simulink model "FX450_model"  (R2019a)
settings: Solver=ode4  StartTime=0.0  StopTime=35  FixedStep=0.001  RelTol=1e-3
PreLoadFcn:
  | filepath  = fileparts(get_param(bdroot, 'FileName'))
  | cd(filepath);
InitFcn:
  | Model_Params;
values from neighbouring files (symbols this model uses):
  aM = 0.478857985732115    (= 0.478857985732)    [Model_Params.m]
  aT = 10.3223    [Model_Params.m]
  bT = 1.7118    [Model_Params.m]
  ModelParam_envAltitude = -50    [Model_Params.m]
  ModelParam_GlobalNoiseGainSwitch = 0.4    [Model_Params.m]
  ModelParam_GPSEphFinal = 0.3    [Model_Params.m]
  ModelParam_GPSEpvFinal = 0.4    [Model_Params.m]
  ModelParam_GPSFix3DFix = 3    [Model_Params.m]
  ModelParam_GPSSatsVisible = 10    [Model_Params.m]
  ModelParam_motorJm = 0    [Model_Params.m]
  ModelParam_noiseBaroCoupleWithSpeed = 0    [Model_Params.m]
  ModelParam_noiseGPSSampTime = 0.2    [Model_Params.m]
  ModelParam_noisePowerIMU = 0    [Model_Params.m]
  ModelParam_noisePowerOffGainAccel = 0.04    [Model_Params.m]
  ModelParam_noisePowerOffGainAccelZ = 0.03    [Model_Params.m]
  ModelParam_noisePowerOffGainGyro = 0.02    [Model_Params.m]
  ModelParam_noisePowerOffGainGyroZ = 0.025    [Model_Params.m]
  ModelParam_noisePowerOffGainMag = 0.02    [Model_Params.m]
  ModelParam_noisePowerOffGainMagZ = 0.035    [Model_Params.m]
  ModelParam_noisePowerOnGainAccel = 0.8    [Model_Params.m]
  ModelParam_noisePowerOnGainAccelZ = 4.5    [Model_Params.m]
  ModelParam_noisePowerOnGainGyro = 2    [Model_Params.m]
  ModelParam_noisePowerOnGainGyroZ = 1    [Model_Params.m]
  ModelParam_noisePowerOnGainMag = 0.025    [Model_Params.m]
  ModelParam_noisePowerOnGainMagZ = 0.05    [Model_Params.m]
  ModelParam_noiseSampleTimeAccel = 0.001    [Model_Params.m]
  ModelParam_noiseSampleTimeGyro = 0.001    [Model_Params.m]
  ModelParam_noiseSampleTimeMag = 0.01    [Model_Params.m]
  ModelParam_noiseUpperGPS = 0.5    [Model_Params.m]
  ModelParam_noiseUpperWindBodyRatio = 0    [Model_Params.m]
  ModelParam_noiseWindSampTime = 0.001    [Model_Params.m]
  ModelParam_timeSampBaro = 0.01    [Model_Params.m]
  ModelParam_uavCCm = [0.0097 0.0085 0.0046]    [Model_Params.m]
  ModelParam_uavCd = [0.2325, 0.2333, 0.5]    [Model_Params.m]
  ModelParam_uavMass = 1.8446    [Model_Params.m]
  ModelParam_uavR = 0.2250    (= 0.225)    [Model_Params.m]
  ModelParam_uavType = int8(3)    [Model_Params.m]
  w1 = -1.813988338293334e+02    (= -181.398833829)    [Model_Params.m]
  w2 = -4.589750663718388e+02    (= -458.975066372)    [Model_Params.m]
  w3 = 1.452124200290536e+03    (= 1452.12420029)    [Model_Params.m]
undefined symbols (not defined in the file or in its folder): Earth, ModelParam_GPSEpvInitial, ModelParam_GPSEpvTimeConstant, ModelParam_noiseLowPassFilterCoeAccel, ModelParam_noiseLowPassFilterCoeGyro, ModelParam_timeSamp, Newton, Raphson, WGS84
libraries: simulink x4, aerolibtransform2 x3, sharedtransform x3, aerolibasang x3, aerolibatmos2 x2, aerolibutil x2, aerolibconvert2 x1, aerolibobsolete x1, shared6dof x1, aerolibnav x1, aerolibgravity2 x1
(part 2 of 2)

== system FX450_model/SensorModel/HILSensorMavModel1/NoiseFilter2 ==
  In1 : Inport
  Demux : Demux  Outputs=3
  Mux1 : Mux  Inputs=3
  Transfer Fcn4 : TransferFcn  Denominator=[0.05 1]
  Transfer Fcn5 : TransferFcn  Denominator=[0.05 1]
  Transfer Fcn6 : TransferFcn  Denominator=[0.05 1]
  Out1 : Outport
  wires:
  Mux1/1 -> Out1/1
  In1/1 -> Demux/1
  Demux/3 -> Transfer Fcn6/1
  Transfer Fcn4/1 -> Mux1/1
  Transfer Fcn6/1 -> Mux1/3
  Demux/1 -> Transfer Fcn4/1
  Transfer Fcn5/1 -> Mux1/2
  Demux/2 -> Transfer Fcn5/1

== matlab function FX450_model/Multicopter_Kinetics&Dynamics/Model_set/Supply Force & Torque ==
  data: uavType input; MotorRads input; R input; Fb output; Mb output; Jm input; Ti input; Mi input; wb input
function [Fb,Mb] = fcn(uavType,MotorRads,R,Jm,Ti,Mi,wb)
% This is control effectiveness model, where Fb is the force produced by motors, Mb is
% the moment produced by motors, and Fd is the resistance produced by the air.
% The gyroscopic torque is not considered here.

% -1: anticlockwise, 1: clockwise 
TypeMotorDirMatrix=[...
    [-1 -1 -1 0 0 0 0 0];... % Tri 3*1 X
    [1 1 1 0 0 0 0 0];...    % Tri 3*1 +
    [-1 -1 1 1 0 0 0 0];... % Quad 4*1 X
    [-1 -1 1 1 0 0 0 0];... % Quad 4*1 +
    [1 -1 1 -1 -1 1 0 0];... % Hex 6*1 X
    [1 -1 1 -1 -1 1 0 0];... % Hex 6*1 +
    [1 -1 1 -1 1 -1 0 0];... % HexCoa 3*2
    [1 1 -1 -1 -1 -1 1 1];... % Oct 8*1 X
    [1 1 -1 -1 -1 -1 1 1];... % Oct 8*1 +
    [-1 1 -1 1 -1 1 -1 1];... % OctCoa 4*2 X
];

TypeMotorAngMatrix=[...
    [pi/3 pi -pi/3 0 0 0 0 0];...
    [pi/3 pi -pi/3 0 0 0 0 0];...
    [pi/4 pi/4+pi pi/4+3*pi/2 pi/4+pi/2 0 0 0 0];...
    [pi/2 3*pi/2 0 pi 0 0 0 0];...
    [pi/2 3/2*pi 3/2*pi+pi/3 pi/2+pi/3 pi/2-pi/3 3/2*pi-pi/3 0 0];...
    [0 pi pi+pi/3 pi/3 -pi/3 pi-pi/3 0 0];...
    [pi/3 pi/3 pi pi -pi/3 -pi/3 0 0];...
    [pi/8 pi+pi/8 pi/8+pi/4 pi-pi/8 -pi/8 3/2*pi-pi/8 3/2*pi+pi/8 pi/2+pi/8];...
    [0 pi pi/4 3/4*pi -pi/4 pi+pi/4 3/2*pi pi/2];...
    [pi/4 -pi/4 pi+pi/4 pi-pi/4 -pi/4 pi/4 pi-pi/4 pi+pi/4];...
];

TypeMotorNonVector=int8([3;3;4;4;6;6;6;8;8;8]);

Mb = [0;0;0];
Fb = [0;0;0];
P=wb(1);Q=wb(2);

if uavType==50
    
    Fb(1)=MotorRads(1)+MotorRads(3);
    Mb(3)=MotorRads(1)*0.1-MotorRads(3)*0.1;
    
    return;
end


if uavType<0||uavType>length(TypeMotorNonVector)
    uavType=int8(1);
end

TypeMotorDirVector=TypeMotorDirMatrix(uavType,:);
TypeMotorAngVector=TypeMotorAngMatrix(uavType,:);

for i=1:TypeMotorNonVector(uavType)
    propAng = TypeMotorAngVector(i);
    propdir = TypeMotorDirVector(i);
    
    % Modified Thrust
    PropT=Ti(i);
    PropM=Mi(i);
    
    %Thrust -> Moment
    Mb=Mb+[-R*sin(propAng)*PropT;R*cos(propAng)*PropT;-PropM*propdir];
    
    %gyroscopic moment
    Mb=Mb+[Q*Jm*MotorRads(i)*propdir;-P*Jm*MotorRads(i)*propdir;0];
    
    Fb=Fb+[0;0;-PropT];
end

 
end

== matlab function FX450_model/Multicopter_Kinetics&Dynamics/Properller Linear-Static Dynamics/MATLAB Function ==
  data: u input; y output; w1 input; w2 input; w3 input
function y = fcn(u,w1,w2,w3)

y = w1*u.^3+w2*u.^2+w3*u;

== matlab function FX450_model/Multicopter_Kinetics&Dynamics/Model_set/Ground Model ==
  settings: updateMethod=DISCRETE
  data: mg input; wb input; Xe input; F1 output; Ve input; M1 output; Quet input; terrainZ input; landed output; takeoff output
function [F1,M1,landed,takeoff] = fcn(mg,wb,Xe,Ve,Quet,terrainZ)
% This is a ground model that can provides reaction force and reaction torque

% persistent z0;
% if isempty(z0)
%      z0=0;
% end

persistent takeoffFlag;
if isempty(takeoffFlag)
     takeoffFlag=int8(0);
end

persistent landFlag;
if isempty(landFlag)
     landFlag=int8(1);
end


z=Xe(3)-terrainZ;

 if (z<-0.3)&&(Ve(3)<-0.1)&&(takeoffFlag<0.5)
    takeoffFlag=int8(1);
    landFlag=int8(0);
 end
 
 if (z>-0.05)&&(Ve(3)>0.1)&&(landFlag<0.5)
    landFlag=int8(1);
    takeoffFlag=int8(0);
    %z0=terrainZ;
 end

takeoff = takeoffFlag;
landed = landFlag;


F1=[0;0;0];
M1=[0;0;0];

if z>=0
%     if z>=0.3
%         if Ve(3)>=5
%             F1(3)=-mg(3)-1000*Ve(3);
%         else
%             F1(3)=-mg(3)-500*z-100*Ve(3);  
%         end
%     elseif z>=0.1
%         if Ve(3)>=2
%             F1(3)=-mg(3)-100*Ve(3);
%         else
%             F1(3)=-mg(3)-50*z-100*Ve(3);  
%         end
%     else
%          if Ve(3)>=1
%             F1(3)=-mg(3)-50*Ve(3);
%         else
%             F1(3)=-mg(3)-5*z-50*Ve(3);  
%         end       
%     end
    if z<0.05
         F1(3)=-mg(3)-10*Ve(3); 
    elseif z<0.1
        F1(3)=-mg(3)-0.5*z-20*Ve(3); 
    else
         F1(3)=-mg(3)-1*z-50*Ve(3); 
    end

    
    F1(1)=-50*Ve(1);
    F1(2)=-50*Ve(2);
    M1=-20*[Quet(2);Quet(3);Quet(4)]-5*wb;
    M1 = M1 * abs(mg(3))*0.0333;
end

== matlab function FX450_model/Multicopter_Kinetics&Dynamics/Model_set/Resistance Force & Torque ==
  data: Vb input; Fd output; Md output; wb input; Cd input; CCm input
function [Fd,Md] = fcn(Vb,wb,Cd, CCm)

Fd =-Cd.*Vb;
 
Md=-CCm.*wb;

 
end

== matlab function FX450_model/SensorModel/HILGPSModel/GenCogVel ==
  data: v output; u input; cot output
function [v,cot] = Ang360(u)
v=norm(u(1:2));

if v < 1
    cot = 0;
else
    cot=atan2d(u(2),u(1));
end
 
if cot<0
    cot=cot+360;
end

== matlab function FX450_model/SensorModel/HILGPSModel/MATLAB Function ==
  data: eph input; FixType output
function FixType = fcn(eph)
if eph <= 2
    FixType=3;
elseif eph <= 4
    FixType=2;
else
    FixType=0;
end

== matlab function FX450_model/Multicopter_Kinetics&Dynamics/Model_set/OnGroundFaceup ==
  data: EulerAng input; y output
function y = fcn(EulerAng)

targetRoll = 0;
% if cos(EulerAng(1))<0
%     targetRoll=pi;  
% end

targetPitch = 0;
% if cos(EulerAng(2))<0
%         targetPitch=pi;
% end
    
y = [targetRoll;targetPitch;EulerAng(3)];

== matlab function FX450_model/SensorModel/HILSensorMavModel1/AccelNoiseGainFunction ==
  data: theta input; Gain output; ModelParam_noisePowerOnGainAccel parameter; ModelParam_noisePowerOffGainAccel parameter; ModelParam_noisePowerOnGainAccelZ parameter; ModelParam_noisePowerOffGainAccelZ parameter
function Gain = fcn(theta, ModelParam_noisePowerOnGainAccel, ModelParam_noisePowerOffGainAccel,ModelParam_noisePowerOnGainAccelZ, ModelParam_noisePowerOffGainAccelZ)
%#codegen
if theta>0.1
Gain = [ModelParam_noisePowerOnGainAccel;ModelParam_noisePowerOnGainAccel;ModelParam_noisePowerOnGainAccelZ];
else
    Gain = [ModelParam_noisePowerOffGainAccel;ModelParam_noisePowerOffGainAccel;ModelParam_noisePowerOffGainAccelZ];
end

== matlab function FX450_model/SensorModel/HILSensorMavModel1/GyroNoiseGainFunction ==
  data: theta input; Gain output; ModelParam_noisePowerOnGainGyro parameter; ModelParam_noisePowerOffGainGyro parameter; ModelParam_noisePowerOnGainGyroZ parameter; ModelParam_noisePowerOffGainGyroZ parameter
function Gain = fcn(theta, ModelParam_noisePowerOnGainGyro, ModelParam_noisePowerOffGainGyro, ModelParam_noisePowerOnGainGyroZ, ModelParam_noisePowerOffGainGyroZ)
%#codegen
if theta>0.1
    Gain = [ModelParam_noisePowerOnGainGyro;ModelParam_noisePowerOnGainGyro;ModelParam_noisePowerOnGainGyroZ];
else
    Gain = [ModelParam_noisePowerOffGainGyro;ModelParam_noisePowerOffGainGyro;ModelParam_noisePowerOffGainGyroZ];
end

== matlab function FX450_model/SensorModel/HILSensorMavModel1/MagNoiseGainFunction ==
  data: theta input; Gain output; ModelParam_noisePowerOnGainMag parameter; ModelParam_noisePowerOffGainMag parameter; ModelParam_noisePowerOnGainMagZ parameter; ModelParam_noisePowerOffGainMagZ parameter
function Gain = fcn(theta, ModelParam_noisePowerOnGainMag, ModelParam_noisePowerOffGainMag, ModelParam_noisePowerOnGainMagZ, ModelParam_noisePowerOffGainMagZ)
%#codegen
if theta>0.1
    Gain = [ModelParam_noisePowerOnGainMag;ModelParam_noisePowerOnGainMag;ModelParam_noisePowerOnGainMagZ];
else
    Gain = [ModelParam_noisePowerOffGainMag;ModelParam_noisePowerOffGainMag;ModelParam_noisePowerOffGainMagZ];
end

== matlab function FX450_model/SensorModel/HILSensorMavModel1/MotorNoiseScaleCoe ==
  data: PWMin input; NoiseScaleCoe output
function NoiseScaleCoe = fcn(PWMin)
%本函数输一个分段函数，分为三段三段斜率不同，具体形状可以通过修改下面四个参数设置

%如何设置合理参数使得噪声在此分段函数前提下更加真实  
%1、首先采集实际飞行过程中飞机的噪声水平然后修改噪声模块的幅值
%2、飞机静止时的噪声则可以通过设置keyPoint1的数值，也就是本分段函数的自变量值为0时候的函数值来调整静止时候飞机传感器噪声

%分段函数有两个起点和转折点，下面四个点一次对应起点两个拐点终点，第一个数表示和坐标的数值，第二个表示对应的函数值
%默认  输入为1是函数值也是1
keyPoint1 = [0 0.05];%不要修改 数字0
keyPoint2 = [0.8 1];
keyPoint3 = [1.7 1];
keyPoint4 = [2 2];%不要修改

%m 范围 0-2 50%油门时候为 m = 1
m = 2*mean(PWMin);
if m <keyPoint2(1)
    NoiseScaleCoe = ((keyPoint2(2) - keyPoint1(2))/(keyPoint2(1)-keyPoint1(1)))*(m - keyPoint1(1)) + keyPoint1(2);
else
    if m > keyPoint2(1) && m < keyPoint3(1)
        NoiseScaleCoe = ((keyPoint3(2) - keyPoint2(2))/(keyPoint3(1)-keyPoint2(1)))*(m - keyPoint2(1)) + keyPoint2(2);
    else
        NoiseScaleCoe = ((keyPoint4(2) - keyPoint3(2))/(keyPoint4(1)-keyPoint3(1)))*(m - keyPoint3(1)) + keyPoint3(2);
    end
end

== matlab function FX450_model/SensorModel/ZLimit ==
  data: zt input; xe input; Xee output
function Xee = fcn(zt,xe)
Xee=xe;
if Xee(3)>zt
    Xee(3)=zt;
end
